simulink model "main"  (R2016a)
settings: Solver=FixedStepAuto  StartTime=0.0  StopTime=inf  FixedStep=0.008  RelTol=1e-3
model workspace: external: MATLAB File initialize_variables_kuramoto.m (data not in the file)
values from neighbouring files (symbols this model uses):
  Angle_offset = [Offset_st, Offset_dev, Offset_rot]    [initialize_variables_kuramoto.m]
  frequency_multiplier = 1    [initialize_variables_kuramoto.m]
  learning_switch = 0    [initialize_variables_matsuoka.m]
  max_dev = 30    [initialize_variables_kuramoto.m]    (also in initialize_variables_matsuoka.m)
  max_rot = 60    [initialize_variables_kuramoto.m]    (also in initialize_variables_matsuoka.m = 90)
  max_stroke = 180    [initialize_variables_kuramoto.m]    (also in initialize_variables_matsuoka.m = 90)
  Offset_st = 0 * gain_st    (= 0)    [initialize_variables_kuramoto.m]
  param_init = [0,0,0,0,0,0 ... (first row only)    [cpg_param_sets.m]    (also in initialize_variables_matsuoka.m)
  param_list = zeros([7,length(Re)*length(A_star)])    [initialize_variables_kuramoto.m]
  step_time = 0.005    [initialize_variables_kuramoto.m]
  w_init = [0 -1.5 0 0 0 0 ... (first row only)    [cpg_param_sets.m]    (also in initialize_variables_matsuoka.m = [0 -2 0 0 -0.1 0)
undefined symbols (not defined in the file or in its folder): frequency, IO3xx, Offset_dev_rot, V
libraries: slrtlib x13, speedgoatlib_fpga x7, simulink x5, powerlib_meascontrol x2
(part 2 of 2)

== matlab function main/Robot/Control/Serial/Read angle1 ==
  data: y input; angle output; old_angle input; old_old_old_angle input; write_type input
function angle  = fcn(y, old_angle,old_old_old_angle, write_type)
%#codegen
angle = nan(1);
angle = old_angle + 0.5*(old_angle-old_old_old_angle);
ID = 1;

for i = 1:1:length(y)-5
    if y(i) == 255 && y(i+1) == 255 && y(i+2) == 253 && y(i+4) == 1 && y(i+5) == 8
        temp = i;       
        Para = y(temp+9:temp+12);
        angle = Position(Para);
    end
end

% if angle == old_angle
%     angle = old_angle + 0.5*(old_angle-old_old_old_angle);    
% end

end

function angle = Position(para)
value_byte = double(typecast(uint8(para),'int32'));
angle = value_byte*360/4095;
end

== matlab function main/Robot/Control/Serial/Read angle2 ==
  data: y input; angle output size=[1 2]; old_angle input; old_old_old_angle input; write_type input
function angle   = fcn(y,old_angle,old_old_old_angle,write_type)
%#codegen

angle = nan(1, 2);
angle_2 = old_angle(1) + 0.5*(old_angle(1)-old_old_old_angle(1));
angle_3 = old_angle(2) + 0.5*(old_angle(2)-old_old_old_angle(2));
ID = [2 3];

for i = 1:1:length(y)-5
    if y(i) == 255 && y(i+1) == 255 && y(i+2) == 253 && y(i+4) == 2 && y(i+5) == 8
        temp_2 = i;
        Para_2 = y(temp_2+9:temp_2+12);
        angle_2 = Position(Para_2);
    elseif y(i) == 255 && y(i+1) == 255 && y(i+2) == 253 && y(i+4) == 3 && y(i+5) == 8
        temp_3 = i;
        Para_3 = y(temp_3+9:temp_3+12);
        angle_3 = Position(Para_3);
    end
end
% 
% if angle_2 == old_angle(1);
%     angle_2 = old_angle(1) + 0.5*(old_angle(1)-old_old_old_angle(1));
% end
% if angle_3 == old_angle(2);
%     angle_3 = old_angle(2) + 0.5*(old_angle(2)-old_old_old_angle(2));
% end

angle = [angle_2 angle_3];

end

function angle = Position(para)
value_byte = double(typecast(uint8(para),'int32'));
angle = value_byte*360/4095;
end

== matlab function main/For data collection/offset_stroke ==
  data: t_old input; offset input; direction input; t_old output; offset output; starting input; starting output; ending input; t input; ending output; collect output; period_cycle input
function [t_old,offset,starting,ending,collect] = offset_update(t_old,offset,direction,starting,ending,t,period_cycle)
%#codegen

% Inputs:
%   t_old = time of last offset change
%   offset = last stroke offset
%   direction = +1 if CCW, -1 if CW
%   starting = whether to assume CPG params are changed started for the
%               first time
%   ending = whether to stop movement/data collection
%   t = current time
%   period_cycle = stroke cycle period

% Outputs:
%   t_old = if new offset is made, then t, else the old t_old
%   offset = offsets for all angles (non-stroke is 0)
%   starting = whether to assume CPG params are changed started for the
%               first time
%   ending = whether to stop movement/data collection
%   collect = 1 if data should be collected, 0 if not

offset_increment = 0 * direction; % deg, how much to move to next location
                                    % MODIFIED TO ONLY STAY AT 0deg
period_cooldown = 3 * period_cycle; % sec, how long to wait after moving to next location to start collecting data
period_cooldown_start = 10 * period_cycle; % sec, how long to wait for the first time after changing CPG params
period_collect = 20 * period_cycle; % sec, how long to collect data for at a location
offset_limits = [0;0]; % deg, min and max value of stroke offset
                        % MODIFIED TO ONLY STAY AT 0deg

collect = 0; % don't collect data by default

if ending == 1 % end data collection
    return;

elseif starting == 1; % if using new CPG params for the first time
    if (t - t_old) >= period_cooldown_start % wait a little more
        % move to next offset location, once cooldown has ended
        t_old = t;
        offset = offset + [offset_increment;0;0];
        starting = 0;
    end
    
elseif (t - t_old) >= (period_cooldown + period_collect) % time to move
    % move to next offset location, once data collection period is over
    t_old = t;
    offset = offset + [offset_increment;0;0];
    
    % end data collection if offset limits are reached
    if offset(1) >= max(offset_limits) || offset(1) <= min(offset_limits);
        ending = 1;
    end

elseif (t - t_old) >= period_cooldown % time to collect data
    collect = 1;

end

== matlab function main/Simulation/QS Model/Quasi-steady model ==
  data: q input; Force output; dq input; ddq input; dt input; Tau output
%%%%%%%%%%%%%%%%%%%%%%%%%%%%%%%%%%%%%%%%%%%%%%%%%%%%%%%%%%%%%%%%%%%%%%%%%%%
%%%%%%%%%%%%%%   Aerodynamic forces and moments calculator   %%%%%%%%%%%%%%
%%%%%%%%%%%%%%%%%%%%%%%%%%%%%%%%%%%%%%%%%%%%%%%%%%%%%%%%%%%%%%%%%%%%%%%%%%%

% This program calcuates the aerodynamic forces and moments generated by a
% flapping wing

% The aerodynamic forces and torques at each wing blade element is
% evaluated by aerodynamics

function [Force,Tau] =Aerodynamic_Force_Torque(q,dq,ddq,dt)
    
% q=[stroke angle;deviation angle; rotation angle]
% dq= dq/dt;
% ddq= dq/dt;

%% Define variables 
    
%     omega_l            % Anular velocity of wing in global frame
%     omega_l_d          % Anular Acc of Right wing in body frame
%     Rcl                %(Rcl* vector_follower=vector_base //    follwer is Wing and Global is base)

    [Rcl,omega_l,omega_l_d] = AngKinZXY(q,dq,ddq);
    %% Hinge parameters

%     lhz  --> Stroke Hinge offset in stroke frame
%     lhx  --> Deviation Hinge offset in deviation frame
%     lhy  --> Rotation Hinge offset in Rotation frame

% Change these parameter according to your setup 
    lhz = [0;0;-0.15];
    lhx = [0;0;0];
    lhy = [0;0.05;0];
    

    vel_h_l = rotz(q(1))*( cross([0;0;dq(1)],lhz) + rotx(q(2))*( cross([dq(2);0;0],lhx) + roty(q(3))*cross([0;dq(3);0],lhy) ));       % Velocity of Hinge in global frame
    
    %% Transform to wing frame
 
    omega_l=Rcl\omega_l;
    omega_l_d=Rcl\omega_l_d;
    vel_h_l  =  Rcl\vel_h_l;
    % transform from global to wing frame



    %%
    rho = 826;      % air density  1.2041(20C) 1.1839(25C)  1.1644(30C)  1.455(35C)
    NumBlade = 10;         % spatial resolution: number of blade elements


% Change these parameter according to your setup 
    Rw = 0.18;          % wing length
    AR = 3;             % Aspect Ratio
    chord = Rw/AR;        % chord length
        

    %% step through a wing span: spanwise location: 0<i<=1
    
    % Initialise variables
    F_t = zeros(3,1);
    Tau_t = zeros(3,1);

    
    for j = 1:NumBlade
        i = j/NumBlade;
        
        % obtain local aerodynamic force/torques in Hinge frame
        % omega_l and omega_r; omega_l_d and omega_r_d in body frame
        % omega_b and vel_h are in global frame
        % omega_b and vel_h have to be expressed differently for left and right wings
        
        % Force and Torque at each blade elements
        [Fi_t, Taui_t] = aerodynamics_left(omega_l,vel_h_l,omega_l_d,i,dt,Rw,chord, NumBlade,rho);

       %% Summation along wing span
       % integrate along wing span and transform to stroke plane frame
       F_t = F_t +  Fi_t;    
       Tau_t =  Tau_t +  Taui_t;


    end

    % All the forces and torque obtain are in Left and Right Wing frame
    % Tranform them to Hinge frame 
 
    Force=Rcl*F_t;

    Tau=Rcl*Tau_t ;
    
end





%% %%%%%%%%%%%%%%%%%%%%%%%%%%%%%%%%%%%%%%%%%%%%%%%%%%%%%%%%%%%%%%%%%%%%%%%%
%  %%%%%%%%%%%%%%%%%%%%%%%%%%%%%%%%%%%%%%%%%%%%%%%%%%%%%%%%%%%%%%%%%%%%%%%%
%  %%%%%%%%%%%%%%%%%%%%%%%%%%%%%%%%%%%%%%%%%%%%%%%%%%%%%%%%%%%%%%%%%%%%%%%%

%-------------------------------------------------------------------
%----------   Aerodynamics Module For Wing  -------------------
%-------------------------------------------------------------------

% This function takes in wing kinematics (angle/velocity/accleration) and body velocity
% and calcuates the aerodynamic force/torque created by each wing blade (w.r.t local blade coordinate frame)
% then convert it to Hinge frame

% torques are with respect to the wing hinges.

% all the values are w.r.t to local blade coordinate frame (different from stroke
% plane frame), except original input of vel_h, omega_w, omege_w_d and omega_b are in stroke plane frame

% wing coordinate frame: (left wing) x points to ventral side (normal to the wing surface), y from wing base to tip, z from trailing to leading edge

% export tip velocity and span-averaged angle of attack

function [Fi, Taui] = aerodynamics_left(omega_w,vel_h, omega_w_d,i,dt,Rw,chord, NumBlade,rho)
 

%% blade-element analysis 
    % i=location of the blade element
    rle = -i*Rw;  % spanwise location of the blade element
    
    % local wing blade velocity 
    vle = cross(omega_w,[0 rle 0]') + vel_h;            % local leading edge velocity in wing frame
    vle(2)=0;                                                   % igonre radial velocity component                                    

    % angular velocity of the last time instant, here omega_b is assumed to be constant
    omega_wLI = omega_w-omega_w_d*dt;
    
    % velocity of the last time instant
    
    vleLI = cross(omega_wLI,[0 rle 0]') + vel_h;                        
    vleLI(2)=0;                                                 % igonre radial velocity component   
    
    % linear accleration along xw direction
    acc_xw = (vle(1)-vleLI(1))/dt;
    % angualr acceleration about yw direction
    omega_yw_dot = omega_w_d(2);

    
    %% Direction of blade velocity
    % get the direction of the local blade velocity
    if norm(vle) ~= 0
        dir_vle = vle/norm(vle)  ;                 % local leading edge velocity direction vector in left wing frame
        alpha = abs(atan(dir_vle(1)/dir_vle(3)));  
    else
        dir_vle = [0;0;0];
        alpha = 0;  
    end
    
    % local drag direction
    dir_drag = -dir_vle;  
    dir_drag(2)=0; 
    % local lift direction
    dir_lift = roty( -sign( vle(1)) *pi/2 ) * dir_vle;         
    % local angle of attack (consider X as imaginary axis and Z as real axis, only 1st and 2nd quadrants are considered)

    %%  wing sectional lift and drag due to translational force components
    % (2*CD(alpha_l)*rle/R) is sectional drag coefficient
    q   = 0.5*rho*(norm(vle))^2;
    FDi = q*(CD_hu(alpha)) * chord * (Rw/NumBlade)*dir_drag;  
    FLi = q*(CL_hu(alpha)) * chord * (Rw/NumBlade)*dir_lift;

    % center of pressure (translational component)
    r_cof_trans = chord*(0.82*abs(alpha)/pi+0.05);

    %%  wing sectional lift and drag due to rotational force components
    
    % Change these parameter according to your setup 
    x_rot = 0.453;  % rotational axis, 0 corresponds to leading edge
    
    Circulation_rot = pi*(0.75-x_rot) * chord^2 * omega_w(2);  % cirulcation over a wing chord
    F_rot_i = (Rw/NumBlade)*[ rho * Circulation_rot * norm(vle), 0, 0]';
    % center of pressure (rotational component)

    r_cof_rot = x_rot*chord;  % old
    
    %%  wing sectional lift and drag due to added-mass force components
    cr = (-x_rot+0.5)*chord; % distance between center of wing rotation and mid-point of wing chord
    % coefficient of virtual mass
    lamda_x = pi*rho*(0.5*chord)^2;
    lamda_xo = -pi*rho*(0.5*chord)^2*cr;

    % added mass force components
    F_addx_i = lamda_x*acc_xw - lamda_xo*omega_yw_dot;

    % force vector due to added mass
    F_add_i = (Rw/NumBlade)*[F_addx_i, 0,0]'; 

    % center of pressure (added mass component)
    r_cof_add = x_rot*chord;   

    %% summation of all force components and convert them to Hinge frame
    % sum  wing local force vectors
    Fi =  (FDi - FLi -F_add_i - F_rot_i);

    % sum wing local torque vectors
    Taui =(cross([0 rle r_cof_trans]',FDi-FLi) + cross([0 rle r_cof_add]',-F_add_i)+cross([0 rle r_cof_rot]',-F_rot_i));  

 

end


function [R,Omega,alpha] = AngKinZXY(q,dq,ddq)

R=rotz(q(1))*rotx(q(2))*roty(q(3));

w2=[0;0;dq(1)] + rotz(q(1)) * ([dq(2);0;0] );
w1=[0;0;dq(1)] ;

Omega=[0;0;dq(1)]...
    + rotz(q(1)) * [dq(2);0;0] ...
    + rotz(q(1)) * rotx(q(2))*[0;dq(3);0];

alpha=[0;0;ddq(1)]...
    + S(w1)*rotz(q(1)) * [dq(2);0;0] +  rotz(q(1)) * [ddq(2);0;0] ...
    + S(w2)*(rotz(q(1)) * rotx(q(2)))*[0;dq(3);0] +(rotz(q(1)) * rotx(q(2)))*[0;ddq(3);0];
end

function Sw = S(w)
%%%%%%%%%%%%%%%%%%%%%%%%%%%%%%%%%%%%%%%%%%%%%%%%%%%%%%%%%%%%%%%%%%%%%%%%%%%
% % Calculate Cross Product matrix
% % cross(w,R)--> Sw  *  R
%%%%%%%%%%%%%%%%%%%%%%%%%%%%%%%%%%%%%%%%%%%%%%%%%%%%%%%%%%%%%%%%%%%%%%%%%%%
Sw = [0 -w(3) w(2);
    w(3) 0 -w(1);
    -w(2) w(1) 0];
end

function CL = CL_hu(alpha)
alphadeg = alpha *180/pi;       % to degrees
CL = 0.245 + 1.63*sin((2.34*alphadeg - 6.3)*pi/180);
end


function CD = CD_hu(alpha)
alphadeg = alpha *180/pi;       % to degrees
CD = 1.88-1.70*cos((2.27*alphadeg - 10.66)*pi/180);
end

== matlab function main/Framework/State calculations/state_find ==
  data: triggers input; ft_meas input; states_old input; ii input; states output; ii output
function [states,ii] = state(triggers,ft_meas,states_old,ii)
%#codegen

states = states_old;

% add up all force measurements in the z and x directions within a cycle
% might have to transform coordinate frame to get them in space frame

% lift
if triggers(1) == 1
    ii(1) = 0; % reset
end
states(1) = (states_old(1) * ii(1) + ft_meas(3)) / (ii(1)+1); % moving avg
ii(1) = ii(1) + 1;

% x
if triggers(2) == 1
    ii(2) = 0; % reset
end
states(2) = (states_old(2) * ii(2) + ft_meas(1)) / (ii(2)+1); % moving avg
ii(2) = ii(2) + 1;

== matlab function main/Framework/State calculations/triggers_find ==
  data: angle_des input; trigger output; angle_des_old input
function trigger = triggers(angle_des, angle_des_old)
%#codegen

% triggers for end of cycle
% if stroke motor angle crosses over the x-axis or if it's at the x-axis,
%   then signify end of cycle. only use the case when it goes from - to +.
if (angle_des_old(1) < 0) && (angle_des(1) >= 0)
    trigger = [1;1];
else
    trigger = [0;0];
end

== matlab function main/Robot/Control/Serial/Write Stroke1 ==
  data: y_stroke output; stroke input; deviation input; rotation input; write_type input; offset_st input; offset_dr input; crc_table input; y_dev_rot output
function [y_stroke, y_dev_rot] = fcn(stroke,deviation,rotation,write_type, offset_st, offset_dr, crc_table)

ID = [1 2 3];


switch write_type
    case 0  % Init
        y_stroke = packetMultiWrite(2,ID,[1 1 1],crc_table)';
        y_dev_rot = packetMultiWrite(2,ID,[1 1 1],crc_table)';
    case 1  % Read
        y_stroke = packetMultiWrite(13,ID(1),[1 1 1],crc_table)';
        y_dev_rot = packetMultiWrite(14,ID,[1 1 1],crc_table)';
    case 2  % Write
        y_stroke = packetMultiWrite(11,ID, [stroke 0 0] + [offset_st 0 0], crc_table)';
        y_dev_rot = packetMultiWrite(11,ID, [0 deviation rotation] + [0 offset_dr], crc_table)';
    otherwise
        y_stroke = packetMultiWrite(11,ID, [stroke 0 0] + [offset_st 0 0], crc_table)';
        y_dev_rot = packetMultiWrite(11,ID, [0 deviation rotation] + [0 offset_dr], crc_table)';
end
end

== matlab function main/For data collection/select_param ==
  data: param_i input; direction input; param_i output; direction output; starting input; ending input; starting output; ending output; ending_all output; param output; param_list input
function [param_i,direction,starting,ending,ending_all,param] = select_param(param_i,direction,starting,ending,param_list)
%#codegen

% Inputs:
%   param_i = index of current parameter set from param_list
%   direction = +1 if CCW, -1 if CW
%   starting = whether to assume CPG params are changed started for the
%               first time
%   ending = whether to stop movement/data collection
%   param_list = matrix with parameter sets in each column

% Outputs:
%   param_i = index of current parameter set from param_list
%   direction = +1 if CCW, -1 if CW
%   starting = whether to assume CPG params are changed started for the
%               first time
%   ending = whether to stop movement/data collection
%   ending_all = true if all parameter sets have been used
%   param = current parameters

N_param = size(param_list,2); % number of CPG parameter sets

param = param_list(:,param_i); % last used CPG parameters
ending_all = false;

% when the previous trajectory has finished collecting data:
if ending == 1
    param_i = param_i + 1;
    
    if param_i > N_param % if all parameter sets have been used up
        ending_all = true;
        return;
    end
    
    param = param_list(:,param_i); % use next CPG parameter set
    
    direction = -1 * direction; % increment offset in opposite direction
    starting = 1; % the other module will make starting = 0 later
    ending = 0;
end
